simulink model "ConstantVelocity"  (R2012b)
settings: Solver=ode2  StartTime=0.0  StopTime=inf  FixedStep=0.001  RelTol=1e-3
undefined symbols (not defined in the file): HIL, LCconv
libraries: quarc_library x5, simulink x3, ScienceStimHasomed_Lib x1
settings Model: SimulationMode=external  ExtModeTrigDuration=500000  Creator=LabUser  LastModifiedBy=LabUser
settings SolverCC: PositivePriorityOrder=on
settings DataIOCC: LimitDataPoints=off
settings RTWCC: SystemTargetFile=quarc_win64.tlc  TemplateMakefile=quarc_default_tmf  Description=QUARC Win64 Target  ProcessScript=quarc_win64_make_rtw_hook
settings STFCustomTargetCC: TargetPreCompLibLocation=C:\PROGRA~3\QUARC\lib\2012b\win64\release  CodeReplacementLibrary=ANSI_C  GeneratePreprocessorConditionals=Disable all  CombineOutputUpdateFcns=on  GRTInterface=off  SystemTargetFile=quarc_win64.tlc
settings GRTTargetCC: TargetPreCompLibLocation=C:\PROGRA~3\QUARC\lib\2012b\win64\release  ParMdlRefBuildCompliant=off  CompOptLevelCompliant=off  ConcurrentExecutionCompliant=off  MatFileLogging=off  ExtMode=on  ExtModeMexFile=quarc_comm

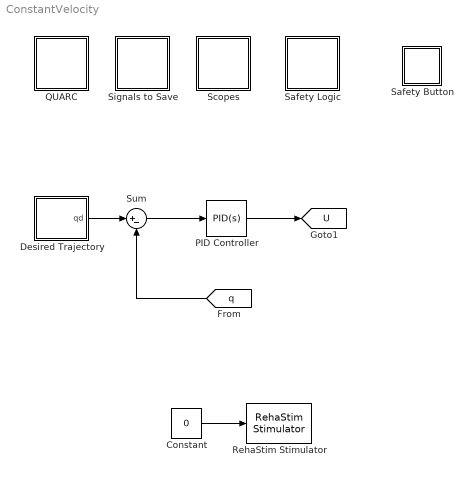
== system ConstantVelocity ==
  Constant : Constant  Value=0
  Desired Trajectory : Subsystem  mask{qmin=-40, qmax=0, vel=10, tau=0.1}
      mask prompts: qmin "Minimum Joint Angle [deg.]:"; qmax "Maximum Joint Angle [deg.]:"; vel "Desired Constant Velocity [deg./s]:"; tau "Smoothing Time Constant [s]:"
  PID Controller : simulink/Continuous/PID Controller  Controller=PID  TimeDomain=Continuous-time  SampleTime=1  IntegratorMethod=Forward Euler  FilterMethod=Forward Euler  Form=Parallel  P=175  I=40  D=1  N=100  InitialConditionSource=internal  InitialConditionForIntegrator=0  InitialConditionForFilter=0  ExternalReset=none  LimitOutput=off  UpperSaturationLimit=inf  LowerSaturationLimit=-inf  LinearizeAsGain=on  AntiWindupMode=none  Kb=1  TrackingMode=off  Kt=1  PParamMin=[]  PParamMax=[]  IParamMin=[]  IParamMax=[]  DParamMin=[]  DParamMax=[]  NParamMin=[]  NParamMax=[]  KbParamMin=[]  KbParamMax=[]  KtParamMin=[]  KtParamMax=[]  POutMin=[]  POutMax=[]  IOutMin=[]  IOutMax=[]  DOutMin=[]  DOutMax=[]  NOutMin=[]  NOutMax=[]  KbOutMin=[]  KbOutMax=[]  KtOutMin=[]  KtOutMax=[]  IntegratorOutMin=[]  IntegratorOutMax=[]  FilterOutMin=[]  FilterOutMax=[]  SumOutMin=[]  SumOutMax=[]  SumI1OutMin=[]  SumI1OutMax=[]  SumI2OutMin=[]  SumI2OutMax=[]  SumI3OutMin=[]  SumI3OutMax=[]  SumDOutMin=[]  SumDOutMax=[]  SaturationOutMin=[]  SaturationOutMax=[]  IntegratorContinuousStateAttributes=''  IntegratorStateMustResolveToSignalObject=off  IntegratorRTWStateStorageClass=Auto  FilterContinuousStateAttributes=''  FilterStateMustResolveToSignalObject=off  FilterRTWStateStorageClass=Auto
  QUARC : Subsystem
  RehaStim Stimulator : ScienceStimHasomed_Lib/RehaStim Stimulator  sFreq=1000  Freq=stimfreq  PWidth=PW
  Safety Button : Subsystem
  Safety Logic : Subsystem  mask{qmin=-50, qmax=10, LClim=60}
      mask prompts: qmin "Minimum Safe Joint Angle [deg.]:"; qmax "Maximum Safe Joint Angle [deg.]:"; LClim "Safe Limit for Load Cell [Nm]:"
      mask help: !!! Don't forget that direction of extension is negative !!!
  Scopes : Subsystem
  Signals to Save : Subsystem
  Sum : Sum  Inputs=|+-
  tag scope: U=global
  wires:
  Constant/1 -> RehaStim Stimulator/1
  Desired Trajectory/1(qd) -> Sum/1
  Sum/1 -> PID Controller/1
  [q] -> Sum/2
  PID Controller/1 -> [U]

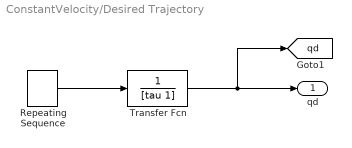
== system ConstantVelocity/Desired Trajectory ==
  Repeating Sequence : simulink/Sources/Repeating Sequence  rep_seq_t=[0 1*vel/(qmax-qmin) 1 1+1*vel/(qmax-qmin) 2]*(qmax-qmin)/vel  rep_seq_y=[qmax qmax qmin qmin qmax]*pi/180
  Transfer Fcn : TransferFcn  Denominator=[tau 1]
  qd : Outport
  tag scope: qd=global
  wires:
  Repeating Sequence/1 -> Transfer Fcn/1
  Transfer Fcn/1 -> [qd], qd/1

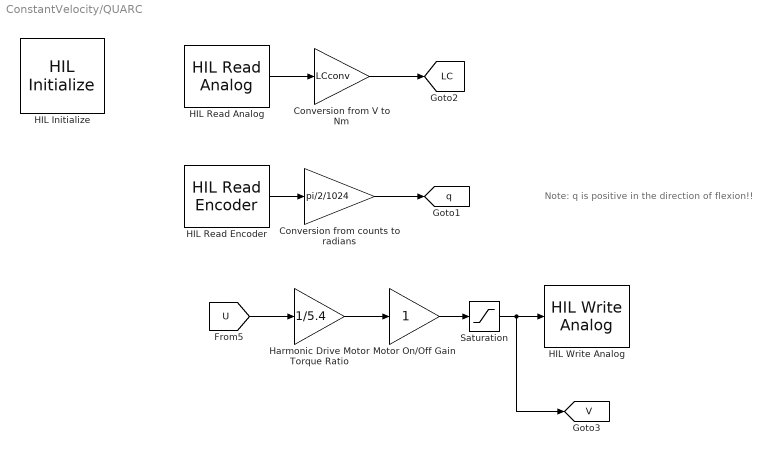
== system ConstantVelocity/QUARC ==
  note: Note: q is positive in the direction of flexion!!
  Conversion from V to Nm : Gain  Gain=LCconv
  Conversion from counts to radians : Gain  Gain=pi/2/1024
  HIL Initialize : quarc_library/Data Acquisition/Generic/Configuration/HIL Initialize  Priority=-99  object_name=HIL-1  board_type=qpid_e  board_number=0  board_options=enc0_dir=0;enc0_filter=1;enc0_a=1;enc0_b=1;enc0_z=0;enc0_reload=0;enc1_dir=0;enc1_filter=1;enc1_a=1;enc1_b=1;enc1_z=0;enc1_reload=0;enc2_dir=0;enc2_filter=1;enc2_a=1;enc2_b=1;enc2_z=0;enc2_reload=0;enc3_dir=0;enc3_filter=1;enc3_a=1;enc3_b=1;enc3_z=0;enc3_reload=0;enc4_dir=0;enc4_filter=1;enc4_a=1;enc4_b=1;enc4_z=0;enc4_reload=0;enc5_dir=0;enc5_filter=1;enc5_a=1;enc5_b=1;enc5_z=0;enc5_reload=0;enc6_dir=0;enc6_filter=1;enc6_a=1;enc6_b=1;enc6_z=0;enc6_reload=0;enc7_dir=0;enc7_filter=1;enc7_a=1;enc7_b=1;enc7_z=0;enc7_reload=0;ext_int_polarity=0;fuse_polarity=0;convert_polarity=0;watchdog_polarity=0;ext_int_watchdog=0;fuse_watchdog=0;trig1_watchdog=0;watchdog_to_trig1=0;watchdog_to_trig2=0;counter_to_trig0=0;trigger_adcs=0;latch_on_adc=0;pwm_immediate=0  exclusive=off  active=off  hardware_clocks=[0:16]  clock_modes=[]  initial_clock_frequencies=[]  set_clock_params_at_start=off  set_clock_params_at_switch_in=off  set_clock_frequencies_at_start=off  set_clock_frequencies_at_switch_in=off  analog_input_channels=[0:7]  analog_input_maximums=10  analog_input_minimums=-10  set_analog_input_params_at_start=off  set_analog_input_params_at_switch_in=off  analog_output_channels=[0:7]  analog_output_maximums=10  analog_output_minimums=-10  initial_analog_outputs=[0]  final_analog_outputs=[0]  watchdog_analog_outputs=0  set_analog_output_params_at_start=off  set_analog_output_params_at_switch_in=off  set_analog_outputs_at_start=on  set_analog_outputs_at_switch_in=off  set_analog_outputs_at_terminate=on  set_analog_outputs_at_switch_out=off  set_analog_outputs_on_watchdog=off  digital_input_channels=[]  digital_output_channels=[]  digital_output_configuration=[]  initial_digital_outputs=[1]  final_digital_outputs=[1]  watchdog_digital_outputs=[2]  set_digital_output_params_at_start=off  set_digital_output_params_at_switch_in=off  set_digital_outputs_at_start=on  set_digital_outputs_at_switch_in=off  set_digital_outputs_at_terminate=on  set_digital_outputs_at_switch_out=off  set_digital_outputs_on_watchdog=off  encoder_channels=[0:7]  quadrature=[4]  encoder_filter_frequency=40e6/1  initial_encoder_counts=[0]  set_encoder_params_at_start=on  set_encoder_params_at_switch_in=off  set_encoder_counts_at_start=off  set_encoder_counts_at_switch_in=off  pwm_channels=[0:7]  pwm_modes=0  pwm_frequency=40e6/4096  pwm_configuration=[0]  pwm_alignment=[0]  pwm_polarity=[1]  pwm_leading_deadband=[0]  pwm_trailing_deadband=[0]  initial_pwm_outputs=[0]  final_pwm_outputs=[0]  watchdog_pwm_outputs=[0]  set_pwm_params_at_start=on  set_pwm_params_at_switch_in=off  set_pwm_outputs_at_start=on  set_pwm_outputs_at_switch_in=off  set_pwm_outputs_at_terminate=on  set_pwm_outputs_at_switch_out=off  set_pwm_outputs_on_watchdog=off  other_output_channels=[]  initial_other_outputs=[]  final_other_outputs=[]  watchdog_other_outputs=[]  set_other_outputs_at_start=off  set_other_outputs_at_switch_in=off  set_other_outputs_at_terminate=off  set_other_outputs_at_switch_out=off  set_other_outputs_on_watchdog=off
  HIL Read Analog : quarc_library/Data Acquisition/Generic/Immediate I//O/HIL Read Analog  object_name=HIL-1  channels=0  sample_time=qc_get_step_size  active=on  vector_output=off
  HIL Read Encoder : quarc_library/Data Acquisition/Generic/Immediate I//O/HIL Read Encoder  object_name=HIL-1  channels=0  sample_time=qc_get_step_size  active=on  vector_output=off  data_type_mode=Inherit via back propagation  data_type=double
  HIL Write Analog : quarc_library/Data Acquisition/Generic/Immediate I//O/HIL Write Analog  object_name=HIL-1  channels=0  sample_time=-1  active=off  vector_input=off
  Harmonic Drive Motor Torque Ratio : Gain  Gain=1/5.4
  Motor On/Off Gain : Gain
  Saturation : Saturate  UpperLimit=10  LowerLimit=-10
  tag scope: LC=global, V=global, q=global
  wires:
  HIL Read Analog/1 -> Conversion from V to Nm/1
  Conversion from counts to radians/1 -> [q]
  Conversion from V to Nm/1 -> [LC]
  HIL Read Encoder/1 -> Conversion from counts to radians/1
  [U] -> Harmonic Drive Motor Torque Ratio/1
  Harmonic Drive Motor Torque Ratio/1 -> Motor On/Off Gain/1
  Motor On/Off Gain/1 -> Saturation/1
  Saturation/1 -> [V], HIL Write Analog/1

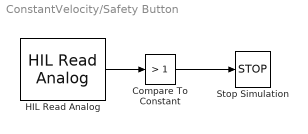
== system ConstantVelocity/Safety Button ==
  Compare To Constant : simulink/Logic and Bit Operations/Compare To Constant  relop=>  const=1  OutDataTypeStr=boolean
  HIL Read Analog : quarc_library/Data Acquisition/Generic/Immediate I//O/HIL Read Analog  object_name=HIL-1  channels=[7]  sample_time=qc_get_step_size  active=on  vector_output=off
  Stop Simulation : Stop
  wires:
  HIL Read Analog/1 -> Compare To Constant/1
  Compare To Constant/1 -> Stop Simulation/1

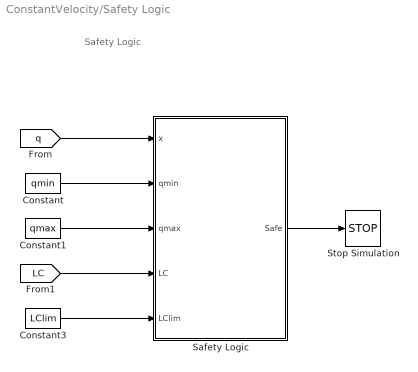
== system ConstantVelocity/Safety Logic ==
  note: Safety Logic
  Constant : Constant  Value=qmin
  Constant1 : Constant  Value=qmax
  Constant3 : Constant  Value=LClim
  Safety Logic : MATLAB Function  TreatAsAtomicUnit=on
  Stop Simulation : Stop
  wires:
  Safety Logic/1(Safe) -> Stop Simulation/1
  [q] -> Safety Logic/1(x)
  Constant/1 -> Safety Logic/2(qmin)
  Constant1/1 -> Safety Logic/3(qmax)
  Constant3/1 -> Safety Logic/5(LClim)
  [LC] -> Safety Logic/4(LC)

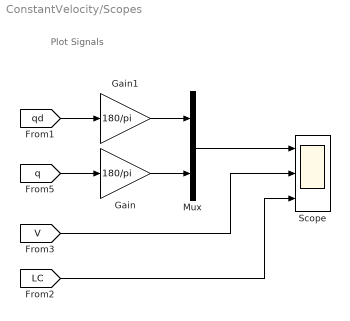
== system ConstantVelocity/Scopes ==
  note: Plot Signals
  Gain : Gain  Gain=180/pi
  Gain1 : Gain  Gain=180/pi
  Mux : Mux  Inputs=2
  Scope : Scope  NumInputPorts=3
      settings: TimeRange=10  YMin=-40~-6.5~3  YMax=0~0.5~8
  wires:
  [q] -> Gain/1
  Mux/1 -> Scope/1
  Gain/1 -> Mux/2
  [qd] -> Gain1/1
  Gain1/1 -> Mux/1
  [LC] -> Scope/3
  [V] -> Scope/2

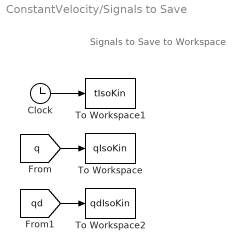
== system ConstantVelocity/Signals to Save ==
  note: Signals to Save to Workspace
  Clock : Clock
  To Workspace : ToWorkspace  VariableName=qIsoKin  SampleTime=-1
  To Workspace1 : ToWorkspace  VariableName=tIsoKin  SampleTime=-1
  To Workspace2 : ToWorkspace  VariableName=qdIsoKin  SampleTime=-1
  wires:
  Clock/1 -> To Workspace1/1
  [q] -> To Workspace/1
  [qd] -> To Workspace2/1

== matlab function ConstantVelocity/Safety Logic/Safety Logic ==
  data: x input; Safe output; qmin input; qmax input; LC input; LClim input
function Safe = fcn(x,qmin,qmax,LC,LClim)

% Outputs Safe=0 when all of the safety criteria are satisfied. If any of
% the safety criteria are not satisfied it will output a 1.

% Initialize vector of safety logic
S = [];

q = x(1)*180/pi;

% Position safety constraint
if (q > qmin) && (q < qmax)
   S = [S 0];
else
    S = [S 1];
end

% Load Cell Safety Constraint
if abs(LC) < LClim
   S = [S 0];
else
    S = [S 1];
end

Safe = any(S);
